simulink model "RigidbodyMPCCurvePathTracking"  (Simulink 8.2)
settings: Solver=ode45  StartTime=0.0  StopTime=40  FixedStep=0.01  RelTol=1e-3
libraries: Solver_SF x1
settings Model: Creator=xuwei  LastModifiedBy=liuho

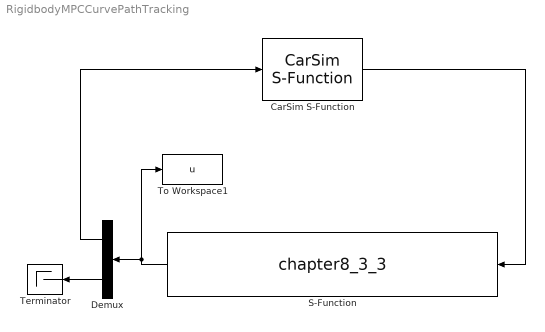
== system RigidbodyMPCCurvePathTracking ==
  CarSim S-Function : Solver_SF/CarSim S-Function  Priority=1  VehicleCode=i_s  SIMFILE=simfile.sim
  Demux : Demux  Outputs=[1 14]
  S-Function : S-Function  FunctionName=chapter8_3_3  EnableBusSupport=off
  Terminator : Terminator
  To Workspace1 : ToWorkspace  VariableName=u  SampleTime=-1  SaveFormat=Structure
  wires:
  CarSim S-Function/1 -> S-Function/1
  S-Function/1 -> Demux/1, To Workspace1/1
  Demux/2 -> Terminator/1
  Demux/1 -> CarSim S-Function/1
